simulink model "Early1"  (Simulink 5.0)
settings: Solver=FixedStepDiscrete  StartTime=0.0  StopTime=10.0  RelTol=1e-3
settings Model: Creator=scaife  LastModifiedBy=scaife  ExtModeAutoUpdateStatusClock=off

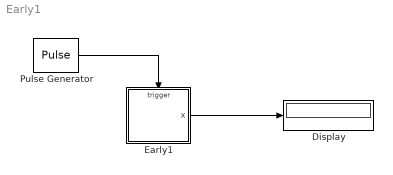
== system Early1 ==
  Display : Display
  Early1 : Stateflow chart
  Pulse Generator : DiscretePulseGenerator
  wires:
  Early1/1(x) -> Display/1
  Pulse Generator/1 -> Early1/Trigger

== stateflow chart Early1 ==
  state A
    state A1/
      en: x=0;
    state A2/
      en: x+=100;
    A1 -> A2 : E{x+=1;}/F;x+=10;
    (default) -> A1
  state B/
    x+=1000;
  (default) -> A
  A -> B : F
  data: x output int32
  events: F local EITHER_EDGE_EVENT; E input EITHER_EDGE_EVENT
